simulink model "Position_Control_Test_SLAM_3LM"  (R2018b)
settings: Solver=VariableStepAuto  StartTime=0.0  StopTime=30  RelTol=1e-3
undefined symbols (not defined in the file): psi, quad, x, y, z
libraries: simulink x7, NLGCToolbox x6, shared6dof x1, aerolibnav x1
settings Model: Creator=hoang  LastModifiedBy=hoang
settings SFSimCC: SimUseLocalCustomCode=off
settings RTWCC: RTWUseLocalCustomCode=off

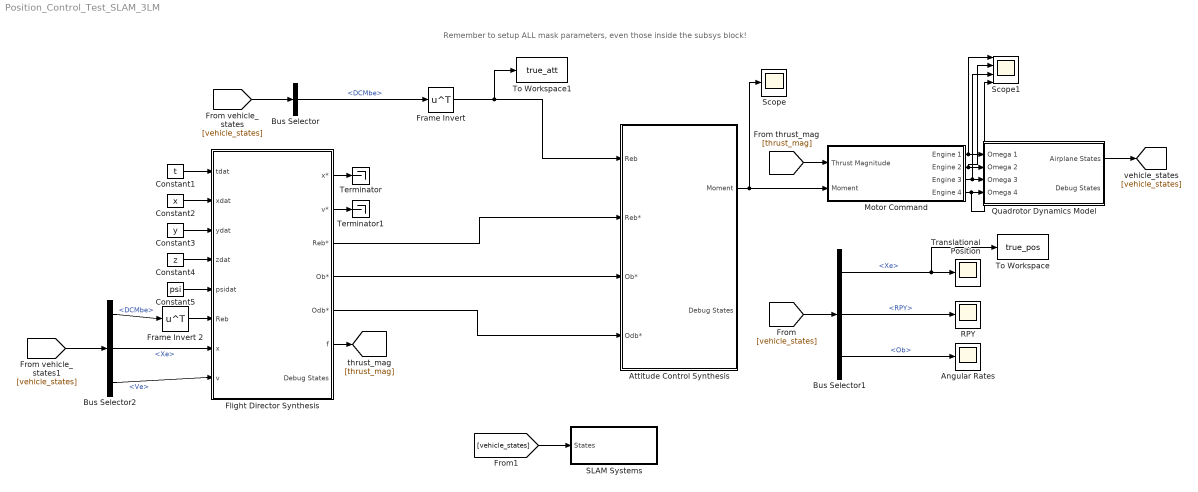
== system Position_Control_Test_SLAM_3LM ==
  note: Remember to setup ALL mask parameters, even those inside the subsys block!
  Angular Rates : Scope
  Attitude Control Synthesis : Subsystem  mask{quadrotor=quad, Ts1=1/120, kr=12, ko=4, Ts=0}
      mask prompts: quadrotor "Quadrotor Parameters"; Ts1 "Sampling Time"; kr "Attitude error gain (Kr)"; ko "Angular velocity error gain (Ko)"; Ts "Sampling Time (Ts)"
      settings: OpenFcn=set_param(gcbh,'LinkStatus','none');
  Bus Selector : BusSelector  OutputSignals=DCMbe
  Bus Selector1 : BusSelector  OutputSignals=Xe,RPY,Ob
  Bus Selector2 : BusSelector  OutputSignals=DCMbe,Xe,Ve
  Constant1 : Constant  Value=t
  Constant2 : Constant  Value=x
  Constant3 : Constant  Value=y
  Constant4 : Constant  Value=z
  Constant5 : Constant  Value=psi
  Flight Director Synthesis : Subsystem  mask{Ts=1/120, kx=64, kv=42, xinit=[0;0;-4], quadrotor=quad}
      mask prompts: Ts "Sampling Time (Ts)"; kx "Position Control Gain (kx)"; kv "Velocity Control Gain (kv)"; xinit "Initial position"; quadrotor "Quadrotor parameters"
      settings: OpenFcn=set_param(gcbh,'LinkStatus','none');
  Frame Invert : Math  Operator=transpose  SaturateOnIntegerOverflow=on
  Frame Invert 2 : Math  Operator=transpose  SaturateOnIntegerOverflow=on
  Motor Command : Subsystem  mask{quadrotor=quad}
      mask prompts: quadrotor "Quadrotor parameters"
      settings: OpenFcn=set_param(gcbh,'LinkStatus','none');
  Quadrotor Dynamics Model : Subsystem  AncestorBlock=NLGCToolbox/Quadrotor Dynamics Model  mask{xinit=[0;0;-4], quadrotor=quad}
      mask prompts: xinit "Initial Position [X,Y,Z]"; quadrotor "Quadrotor Model Struct"
  RPY : Scope
  SLAM Systems : Subsystem
  Scope : Scope
  Scope1 : Scope  NumInputPorts=4
  Terminator : Terminator
  Terminator1 : Terminator
  To Workspace : ToWorkspace  VariableName=true_pos  SaveFormat=Timeseries  SampleTime=-1
  To Workspace1 : ToWorkspace  VariableName=true_att  SaveFormat=Timeseries  SampleTime=-1
  Translational Position : Scope
  wires:
  Motor Command/1(Engine 1) -> Scope1/1, Quadrotor Dynamics Model/1(Omega 1)
  Motor Command/2(Engine 2) -> Scope1/2, Quadrotor Dynamics Model/2(Omega 2)
  Motor Command/3(Engine 3) -> Scope1/3, Quadrotor Dynamics Model/3(Omega 3)
  Motor Command/4(Engine 4) -> Scope1/4, Quadrotor Dynamics Model/4(Omega 4)
  Quadrotor Dynamics Model/1(Airplane States) -> [vehicle_states]
  [vehicle_states] -> Bus Selector/1
  Bus Selector/1 -> Frame Invert/1  "<DCMbe>"
  Frame Invert/1 -> To Workspace1/1, Attitude Control Synthesis/1(Reb)
  Flight Director Synthesis/3(Reb*) -> Attitude Control Synthesis/2(Reb*)
  Flight Director Synthesis/4(Ob*) -> Attitude Control Synthesis/3(Ob*)
  [vehicle_states] -> Bus Selector1/1
  Bus Selector1/2 -> RPY/1  "<RPY>"
  Bus Selector1/3 -> Angular Rates/1  "<Ob>"
  Bus Selector1/1 -> To Workspace/1, Translational Position/1  "<Xe>"
  Attitude Control Synthesis/1(Moment) -> Scope/1, Motor Command/2(Moment)
  Constant1/1 -> Flight Director Synthesis/1(tdat)
  Constant2/1 -> Flight Director Synthesis/2(xdat)
  Constant3/1 -> Flight Director Synthesis/3(ydat)
  Constant4/1 -> Flight Director Synthesis/4(zdat)
  Constant5/1 -> Flight Director Synthesis/5(psidat)
  [vehicle_states] -> Bus Selector2/1
  Frame Invert 2/1 -> Flight Director Synthesis/6(Reb)
  Bus Selector2/1 -> Frame Invert 2/1  "<DCMbe>"
  Bus Selector2/2 -> Flight Director Synthesis/7(x)  "<Xe>"
  Bus Selector2/3 -> Flight Director Synthesis/8(v)  "<Ve>"
  Flight Director Synthesis/5(Odb*) -> Attitude Control Synthesis/4(Odb*)
  Flight Director Synthesis/1(x*) -> Terminator/1
  Flight Director Synthesis/2(v*) -> Terminator1/1
  Flight Director Synthesis/6(f) -> [thrust_mag]
  [thrust_mag] -> Motor Command/1(" Thrust Magnitude")
  [vehicle_states] -> SLAM Systems/1(States)

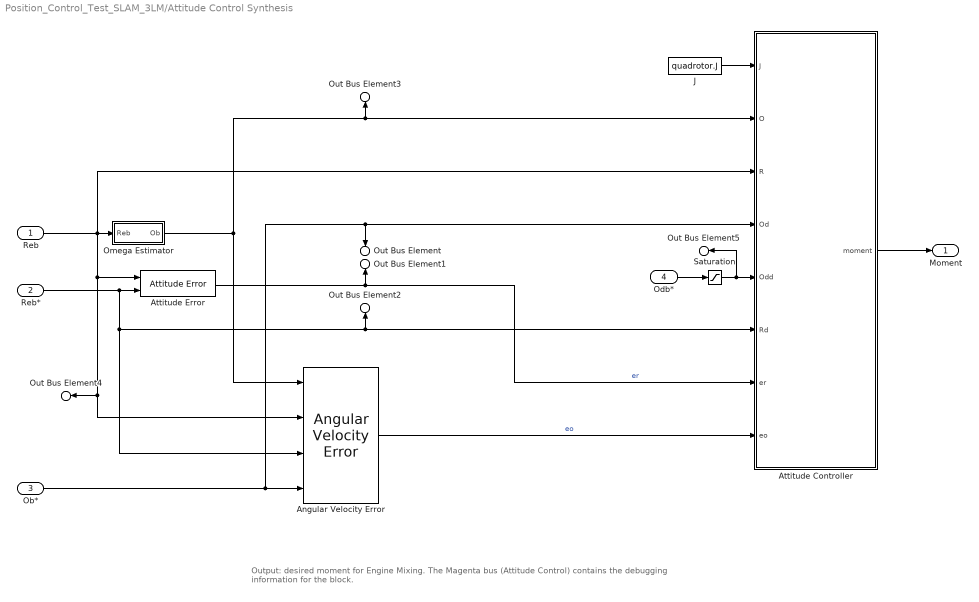
== system Position_Control_Test_SLAM_3LM/Attitude Control Synthesis ==
  note: Output: desired moment for Engine Mixing. The Magenta bus (Attitude Control) contains the debugging information for the block.
  Reb : Inport
  Reb* : Inport  Port=2
  Ob* : Inport  Port=3
  Odb* : Inport  Port=4
  Angular Velocity Error : NLGCToolbox/Angular Velocity Error  SystemSampleTime=-1
      settings: SourceProductName=Thinh - NLGC for Quadrotor
  Attitude Controller : MATLAB Function  TreatAsAtomicUnit=on
  Attitude Error : NLGCToolbox/Attitude Error  SystemSampleTime=-1
      settings: SourceProductName=Thinh - NLGC for Quadrotor
  J : Constant  Value=quadrotor.J
  Omega Estimator : Subsystem  mask{Ts=Ts1}
      mask prompts: Ts "Sampling Time (Ts)"
      settings: OpenFcn=set_param(gcbh,'LinkStatus','none');
  Saturation : Saturate  UpperLimit=1  LowerLimit=-1
  Moment : Outport
  Out Bus Element : Outport  Port=2  PortName=Debug States  Element=Ob*
  Out Bus Element1 : Outport  Port=2  PortName=Debug States  Element=er
  Out Bus Element2 : Outport  Port=2  PortName=Debug States  Element=Reb*
  Out Bus Element3 : Outport  Port=2  PortName=Debug States  Element=Ob
  Out Bus Element4 : Outport  Port=2  PortName=Debug States  Element=Reb
  Out Bus Element5 : Outport  Port=2  PortName=Debug States  Element=Odb*
  wires:
  Attitude Error/1 -> Out Bus Element1/1, Attitude Controller/7(er)  "er"
  Omega Estimator/1(Ob) -> Angular Velocity Error/1, Out Bus Element3/1, Attitude Controller/2(O)
  Angular Velocity Error/1 -> Attitude Controller/8(eo)  "eo"
  Saturation/1 -> Attitude Controller/5(Odd), Out Bus Element5/1
  Ob*/1 -> Angular Velocity Error/4, Attitude Controller/4(Od), Out Bus Element/1
  Reb*/1 -> Attitude Error/2, Angular Velocity Error/3, Attitude Controller/6(Rd), Out Bus Element2/1
  J/1 -> Attitude Controller/1(J)
  Attitude Controller/1(moment) -> Moment/1
  Odb*/1 -> Saturation/1
  Reb/1 -> Omega Estimator/1(Reb), Attitude Error/1, Angular Velocity Error/2, Out Bus Element4/1, Attitude Controller/3(R)

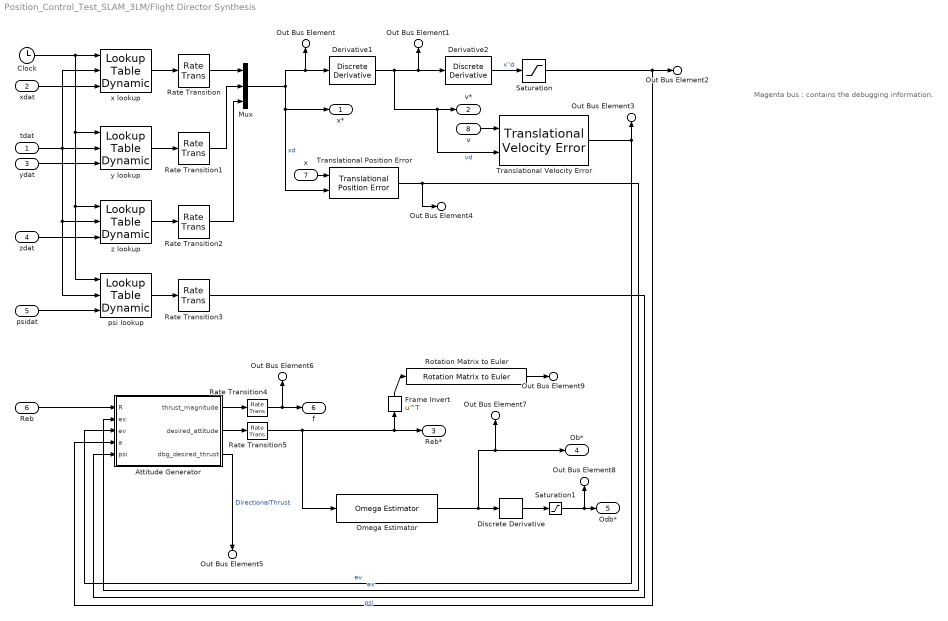
== system Position_Control_Test_SLAM_3LM/Flight Director Synthesis ==
  note: Magenta bus : contains the debugging information.
  tdat : Inport
  xdat : Inport  Port=2
  ydat : Inport  Port=3
  zdat : Inport  Port=4
  psidat : Inport  Port=5
  Reb : Inport  Port=6
  x : Inport  Port=7
  v : Inport  Port=8
  Attitude Generator : MATLAB Function  TreatAsAtomicUnit=on
  Clock : Clock
  Derivative1 : simulink/Discrete/Discrete Derivative  gainval=1.0  ICPrevScaledInput=xinit/Ts  OutMin=[]  OutMax=[]  OutDataType=fixdt(1, 16)  OutScaling=2^-10  DoSatur=off
  Derivative2 : simulink/Discrete/Discrete Derivative  gainval=1.0  ICPrevScaledInput=0.0  OutMin=[]  OutMax=[]  OutDataType=fixdt(1, 16)  OutScaling=2^-10  DoSatur=off
  Discrete Derivative : simulink/Discrete/Discrete Derivative  gainval=1.0  ICPrevScaledInput=0.0  OutMin=[]  OutMax=[]  OutDataType=fixdt(1, 16)  OutScaling=2^-10  DoSatur=off
  Frame Invert : Math  Operator=transpose  SaturateOnIntegerOverflow=on
  Mux : Mux  Inputs=3
  Omega Estimator : NLGCToolbox/Omega Estimator  Ts=Ts
      settings: SourceProductName=Thinh - NLGC for Quadrotor
  Rate Transition{,1..5} (6 alike) : RateTransition  OutPortSampleTime=Ts
  Rotation Matrix to Euler : NLGCToolbox/Rotation Matrix to Euler  SystemSampleTime=-1
      settings: SourceProductName=Thinh - NLGC for Quadrotor
  Saturation : Saturate  UpperLimit=1  LowerLimit=-1
  Saturation1 : Saturate  UpperLimit=1  LowerLimit=-1
  Translational Position Error : NLGCToolbox/Translational Position Error  SystemSampleTime=-1
      settings: SourceProductName=Thinh - NLGC for Quadrotor
  Translational Velocity Error : NLGCToolbox/Translational Velocity Error  SystemSampleTime=-1
      settings: SourceProductName=Thinh - NLGC for Quadrotor
  psi lookup : simulink/Lookup Tables/Lookup Table Dynamic  LookUpMeth=Interpolation-Use End Values  OutDataType=fixdt('double')  OutScaling=[]  OutputDataTypeScalingMode=Specify via dialog  OutDataTypeStr=double  DoSatur=off
      settings: SourceProductName=Simulink
  x lookup : simulink/Lookup Tables/Lookup Table Dynamic  LookUpMeth=Interpolation-Use End Values  OutDataType=fixdt('double')  OutScaling=[]  OutputDataTypeScalingMode=Specify via dialog  OutDataTypeStr=double  DoSatur=off
      settings: SourceProductName=Simulink
  y lookup : simulink/Lookup Tables/Lookup Table Dynamic  LookUpMeth=Interpolation-Use End Values  OutDataType=fixdt('double')  OutScaling=[]  OutputDataTypeScalingMode=Specify via dialog  OutDataTypeStr=double  DoSatur=off
      settings: SourceProductName=Simulink
  z lookup : simulink/Lookup Tables/Lookup Table Dynamic  LookUpMeth=Interpolation-Use End Values  OutDataType=fixdt('double')  OutScaling=[]  OutputDataTypeScalingMode=Specify via dialog  OutDataTypeStr=double  DoSatur=off
      settings: SourceProductName=Simulink
  x* : Outport
  v* : Outport  Port=2
  Reb* : Outport  Port=3
  Ob* : Outport  Port=4
  Odb* : Outport  Port=5
  f : Outport  Port=6
  Out Bus Element : Outport  Port=7  PortName=Debug States  Element=xd
  Out Bus Element1 : Outport  Port=7  PortName=Debug States  Element=vd
  Out Bus Element2 : Outport  Port=7  PortName=Debug States  Element=x''d
  Out Bus Element3 : Outport  Port=7  PortName=Debug States  Element=ev
  Out Bus Element4 : Outport  Port=7  PortName=Debug States  Element=ex
  Out Bus Element5 : Outport  Port=7  PortName=Debug States  Element=DirectionalThrust
  Out Bus Element6 : Outport  Port=7  PortName=Debug States  Element=DesiredThrust
  Out Bus Element7 : Outport  Port=7  PortName=Debug States  Element=DesiredOmega
  Out Bus Element8 : Outport  Port=7  PortName=Debug States  Element=Desired Angular Acceleration
  Out Bus Element9 : Outport  Port=7  PortName=Debug States  Element=RPY*
  wires:
  Frame Invert/1 -> Rotation Matrix to Euler/1
  Rotation Matrix to Euler/1 -> Out Bus Element9/1
  Saturation1/1 -> Out Bus Element8/1, Odb*/1
  Attitude Generator/3(dbg_desired_thrust) -> Out Bus Element5/1  "DirectionalThrust"
  Omega Estimator/1 -> Out Bus Element7/1, Ob*/1, Discrete Derivative/1
  v/1 -> Translational Velocity Error/1
  psidat/1 -> psi lookup/3
  Translational Velocity Error/1 -> Out Bus Element3/1, Attitude Generator/3(ev)  "ev"
  Translational Position Error/1 -> Attitude Generator/2(ex), Out Bus Element4/1  "ex"
  x/1 -> Translational Position Error/1
  Mux/1 -> Out Bus Element/1, Derivative1/1, Translational Position Error/2, x*/1  "xd"
  Rate Transition4/1 -> Out Bus Element6/1, f/1
  Rate Transition5/1 -> Frame Invert/1, Reb*/1, Omega Estimator/1
  Discrete Derivative/1 -> Saturation1/1
  Reb/1 -> Attitude Generator/1(R)
  Attitude Generator/2(desired_attitude) -> Rate Transition5/1
  Attitude Generator/1(thrust_magnitude) -> Rate Transition4/1
  Rate Transition3/1 -> Attitude Generator/5(psi)  "psi"
  Derivative2/1 -> Saturation/1  "x''d"
  psi lookup/1 -> Rate Transition3/1
  Derivative1/1 -> v*/1, Translational Velocity Error/2, Out Bus Element1/1, Derivative2/1  "vd"
  Rate Transition2/1 -> Mux/3
  Rate Transition1/1 -> Mux/2
  Rate Transition/1 -> Mux/1
  z lookup/1 -> Rate Transition2/1
  y lookup/1 -> Rate Transition1/1
  x lookup/1 -> Rate Transition/1
  zdat/1 -> z lookup/3
  ydat/1 -> y lookup/3
  xdat/1 -> x lookup/3
  Clock/1 -> x lookup/1, y lookup/1, z lookup/1, psi lookup/1
  tdat/1 -> y lookup/2, x lookup/2, z lookup/2, psi lookup/2
  Saturation/1 -> Attitude Generator/4(a), Out Bus Element2/1

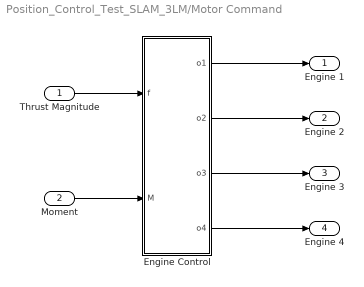
== system Position_Control_Test_SLAM_3LM/Motor Command ==
  " Thrust Magnitude" : Inport
  Moment : Inport  Port=2
  Engine Control : MATLAB Function  TreatAsAtomicUnit=on
  Engine 1 : Outport
  Engine 2 : Outport  Port=2
  Engine 3 : Outport  Port=3
  Engine 4 : Outport  Port=4
  wires:
  Engine Control/4(o4) -> Engine 4/1
  Engine Control/3(o3) -> Engine 3/1
  Engine Control/2(o2) -> Engine 2/1
  Engine Control/1(o1) -> Engine 1/1
  Moment/1 -> Engine Control/2(M)
  " Thrust Magnitude"/1 -> Engine Control/1(f)

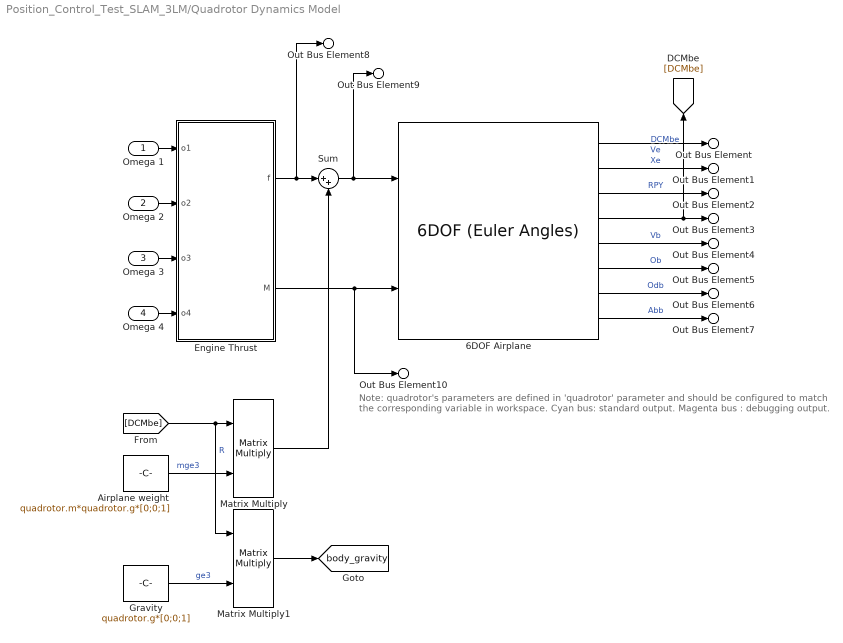
== system Position_Control_Test_SLAM_3LM/Quadrotor Dynamics Model ==
  note: Note: quadrotor's parameters are defined in 'quadrotor' parameter and should be configured to match the corresponding variable in workspace.
      | Cyan bus: standard output.
      | Magenta bus : debugging output.
  Omega 1 : Inport
  Omega 2 : Inport  Port=2
  Omega 3 : Inport  Port=3
  Omega 4 : Inport  Port=4
  6DOF Airplane : shared6dof/6DOF (Euler Angles)  units=Metric (MKS)  mtype=Fixed  rep=Euler Angles  xme_0=xinit  Vm_0=[0 0 0]  eul_0=[0 0 0]  pm_0=[0 0 0]  mass_0=quad.m  mass_e=0.5  mass_f=2.0  inertia=quad.J  inertia_e=eye(3)  inertia_f=2*eye(3)  k_quat=1.0  vre_flag=on  abi_flag=off  aMode=aMode  xme_statename=''  Vm_statename=''  eul_statename=''  quat_statename=''  pm_statename=''  mass_statename=''
      settings: SourceProductBaseCode=AE
  Airplane weight : Constant  Value=quadrotor.m*quadrotor.g*[0;0;1]
  Engine Thrust : MATLAB Function  TreatAsAtomicUnit=on
  Gravity : Constant  Value=quadrotor.g*[0;0;1]
  Matrix Multiply : Product  Multiplication=Matrix(*)
  Matrix Multiply1 : Product  Multiplication=Matrix(*)
  Sum : Sum  Inputs=|++
  Out Bus Element : Outport  PortName=Airplane States  Element=Ve
  Out Bus Element1 : Outport  PortName=Airplane States  Element=Xe
  Out Bus Element2 : Outport  PortName=Airplane States  Element=RPY
  Out Bus Element3 : Outport  PortName=Airplane States  Element=DCMbe
  Out Bus Element4 : Outport  PortName=Airplane States  Element=Vb
  Out Bus Element5 : Outport  PortName=Airplane States  Element=Ob
  Out Bus Element6 : Outport  PortName=Airplane States  Element=Odb
  Out Bus Element7 : Outport  PortName=Airplane States  Element=Abb
  Out Bus Element8 : Outport  Port=2  PortName=Debug States  Element=Thrust
  Out Bus Element9 : Outport  Port=2  PortName=Debug States  Element=Total Force
  Out Bus Element10 : Outport  Port=2  PortName=Debug States  Element=Moment
  tag scope: body_gravity=global
  wires:
  [DCMbe] -> Matrix Multiply1/1, Matrix Multiply/1  "R"
  Omega 1/1 -> Engine Thrust/1(o1)
  Omega 4/1 -> Engine Thrust/4(o4)
  Omega 3/1 -> Engine Thrust/3(o3)
  Omega 2/1 -> Engine Thrust/2(o2)
  Sum/1 -> 6DOF Airplane/1, Out Bus Element9/1
  Engine Thrust/2(M) -> 6DOF Airplane/2, Out Bus Element10/1
  6DOF Airplane/8 -> Out Bus Element7/1  "Abb"
  6DOF Airplane/5 -> Out Bus Element4/1  "Vb"
  6DOF Airplane/7 -> Out Bus Element6/1  "Odb"
  6DOF Airplane/2 -> Out Bus Element1/1  "Xe"
  6DOF Airplane/4 -> [DCMbe], Out Bus Element3/1  "DCMbe"
  6DOF Airplane/3 -> Out Bus Element2/1  "RPY"
  6DOF Airplane/1 -> Out Bus Element/1  "Ve"
  Matrix Multiply/1 -> Sum/2
  Engine Thrust/1(f) -> Sum/1, Out Bus Element8/1
  Airplane weight/1 -> Matrix Multiply/2  "mge3"
  6DOF Airplane/6 -> Out Bus Element5/1  "Ob"
  Gravity/1 -> Matrix Multiply1/2  "ge3"
  Matrix Multiply1/1 -> [body_gravity]

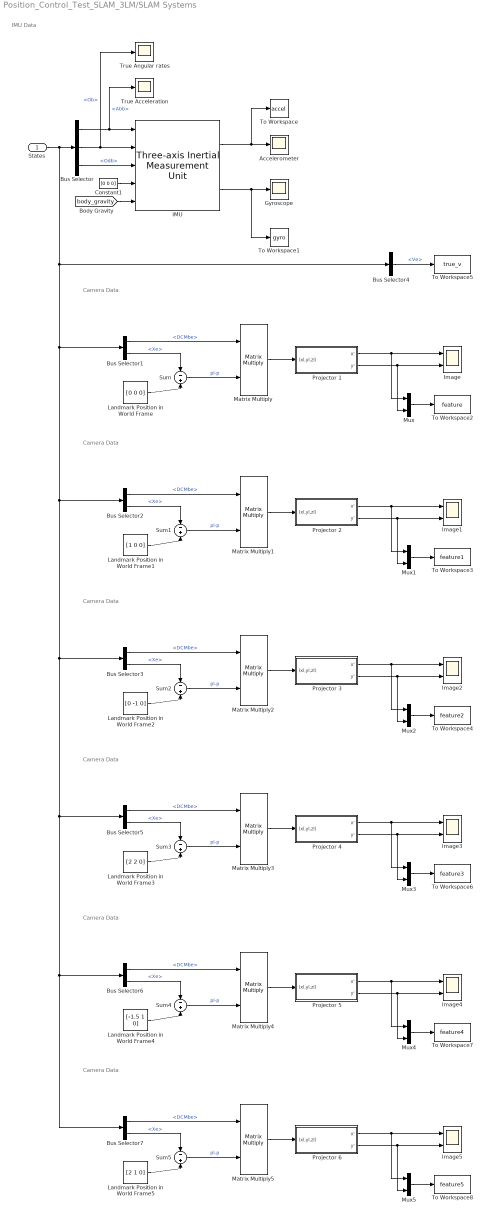
== system Position_Control_Test_SLAM_3LM/SLAM Systems ==
  note: Camera Data
  note: IMU Data
  note: Camera Data
  note: Camera Data
  note: Camera Data
  note: Camera Data
  note: Camera Data
  States : Inport
  Accelerometer : Scope
  Bus Selector : BusSelector  OutputSignals=Abb,Ob,Odb
  Bus Selector{1..3,5..7} (6 alike) : BusSelector  OutputSignals=DCMbe,Xe
  Bus Selector4 : BusSelector  OutputSignals=Ve
  Constant1 : Constant  Value=[0 0 0]
  Gyroscope : Scope
  IMU : aerolibnav/Three-axis Inertial Measurement Unit  units=Metric (MKS)  imu=[0 0 0]  i_Ts=0  dtype_a=off  w_a=190  z_a=0.707  a_sf_cc=[1 0 0; 0 1 0; 0 0 1]  a_bias=[0 0 0]  a_sat="[-inf  -inf  -inf  inf inf inf]"  dtype_g=off  w_g=190  z_g=0.707  g_sf_cc=[1 0 0; 0 1 0; 0 0 1]  g_bias=[0 0 0]  g_sens=[0 0 0]  g_sat="[-inf  -inf  -inf  inf inf inf]"  i_rand=off  i_seeds=[23093 23094 23095 23096 23097 23098]  i_pow=[0.001 0.001 0.001 0.0001 0.0001 0.0001]
  Image{,1..5} (6 alike) : Scope  NumInputPorts=2
  Landmark Position in World Frame : Constant  Value=[0 0 0]
  Landmark Position in World Frame1 : Constant  Value=[1 0 0]
  Landmark Position in World Frame2 : Constant  Value=[0 -1 0]
  Landmark Position in World Frame3 : Constant  Value=[2 2 0]
  Landmark Position in World Frame4 : Constant  Value=[-1.5 1 0]
  Landmark Position in World Frame5 : Constant  Value=[2 1 0]
  Matrix Multiply{,1..5} (6 alike) : Product  Multiplication=Matrix(*)
  Mux{,1..5} (6 alike) : Mux  Inputs=2
  Projector 1 : Subsystem
  Projector 2 : Subsystem
  Projector 3 : Subsystem
  Projector 4 : Subsystem
  Projector 5 : Subsystem
  Projector 6 : Subsystem
  Sum{,1..5} (6 alike) : Sum  Inputs=-+
  To Workspace : ToWorkspace  VariableName=accel  SaveFormat=Timeseries  SampleTime=-1
  To Workspace1 : ToWorkspace  VariableName=gyro  SaveFormat=Timeseries  SampleTime=-1
  To Workspace2 : ToWorkspace  VariableName=feature  SaveFormat=Timeseries  SampleTime=-1
  To Workspace3 : ToWorkspace  VariableName=feature1  SaveFormat=Timeseries  SampleTime=-1
  To Workspace4 : ToWorkspace  VariableName=feature2  SaveFormat=Timeseries  SampleTime=-1
  To Workspace5 : ToWorkspace  VariableName=true_v  SaveFormat=Timeseries  SampleTime=-1
  To Workspace6 : ToWorkspace  VariableName=feature3  SaveFormat=Timeseries  SampleTime=-1
  To Workspace7 : ToWorkspace  VariableName=feature4  SaveFormat=Timeseries  SampleTime=-1
  To Workspace8 : ToWorkspace  VariableName=feature5  SaveFormat=Timeseries  SampleTime=-1
  True Acceleration : Scope
  True Angular rates : Scope
  wires:
  Bus Selector/2 -> True Angular rates/1, IMU/2  "<Ob>"
  Bus Selector/3 -> IMU/3  "<Odb>"
  Bus Selector/1 -> True Acceleration/1, IMU/1  "<Abb>"
  IMU/1 -> To Workspace/1, Accelerometer/1
  Constant1/1 -> IMU/4
  IMU/2 -> To Workspace1/1, Gyroscope/1
  [body_gravity] -> IMU/5
  Bus Selector1/1 -> Matrix Multiply/1  "<DCMbe>"
  Landmark Position in World Frame/1 -> Sum/2
  Bus Selector1/2 -> Sum/1  "<Xe>"
  Sum/1 -> Matrix Multiply/2  "pl-p"
  Matrix Multiply/1 -> Projector 1/1((xl,yl,zl))
  Projector 1/2(y') -> Mux/2, Image/2
  Projector 1/1(x') -> Mux/1, Image/1
  Mux/1 -> To Workspace2/1
  Matrix Multiply1/1 -> Projector 2/1((xl,yl,zl))
  Landmark Position in World Frame1/1 -> Sum1/2
  Bus Selector2/1 -> Matrix Multiply1/1  "<DCMbe>"
  Projector 2/1(x') -> Mux1/1, Image1/1
  Mux1/1 -> To Workspace3/1
  Bus Selector2/2 -> Sum1/1  "<Xe>"
  Sum1/1 -> Matrix Multiply1/2  "pl-p"
  Projector 2/2(y') -> Mux1/2, Image1/2
  Projector 3/2(y') -> Image2/2, Mux2/2
  Sum2/1 -> Matrix Multiply2/2  "pl-p"
  Bus Selector3/2 -> Sum2/1  "<Xe>"
  Mux2/1 -> To Workspace4/1
  Projector 3/1(x') -> Image2/1, Mux2/1
  Bus Selector3/1 -> Matrix Multiply2/1  "<DCMbe>"
  Landmark Position in World Frame2/1 -> Sum2/2
  Matrix Multiply2/1 -> Projector 3/1((xl,yl,zl))
  Bus Selector4/1 -> To Workspace5/1  "<Ve>"
  Matrix Multiply3/1 -> Projector 4/1((xl,yl,zl))
  Landmark Position in World Frame3/1 -> Sum3/2
  Bus Selector5/1 -> Matrix Multiply3/1  "<DCMbe>"
  Projector 4/1(x') -> Mux3/1, Image3/1
  Mux3/1 -> To Workspace6/1
  Bus Selector5/2 -> Sum3/1  "<Xe>"
  Sum3/1 -> Matrix Multiply3/2  "pl-p"
  Projector 4/2(y') -> Mux3/2, Image3/2
  Projector 5/2(y') -> Image4/2, Mux4/2
  Sum4/1 -> Matrix Multiply4/2  "pl-p"
  Bus Selector6/2 -> Sum4/1  "<Xe>"
  Mux4/1 -> To Workspace7/1
  Projector 5/1(x') -> Image4/1, Mux4/1
  Bus Selector6/1 -> Matrix Multiply4/1  "<DCMbe>"
  Landmark Position in World Frame4/1 -> Sum4/2
  Matrix Multiply4/1 -> Projector 5/1((xl,yl,zl))
  Matrix Multiply5/1 -> Projector 6/1((xl,yl,zl))
  Landmark Position in World Frame5/1 -> Sum5/2
  Bus Selector7/1 -> Matrix Multiply5/1  "<DCMbe>"
  Projector 6/1(x') -> Mux5/1, Image5/1
  Mux5/1 -> To Workspace8/1
  Bus Selector7/2 -> Sum5/1  "<Xe>"
  Sum5/1 -> Matrix Multiply5/2  "pl-p"
  Projector 6/2(y') -> Mux5/2, Image5/2
  States/1 -> Bus Selector4/1, Bus Selector7/1, Bus Selector6/1, Bus Selector5/1, Bus Selector3/1, Bus Selector2/1, Bus Selector1/1, Bus Selector/1

== system Position_Control_Test_SLAM_3LM/Attitude Control Synthesis/Omega Estimator ==
  Reb : Inport
  Delay : Delay  DelayLength=1
  Omega Estimator : MATLAB Function  TreatAsAtomicUnit=on
  Rate Transition2 : RateTransition  InitialCondition=diag([1,1,1])  OutPortSampleTime=Ts
  Ob : Outport
  wires:
  Delay/1 -> Omega Estimator/1(Rd1)
  Reb/1 -> Rate Transition2/1
  Omega Estimator/1(Omega) -> Ob/1
  Rate Transition2/1 -> Delay/1, Omega Estimator/2(Rd2)

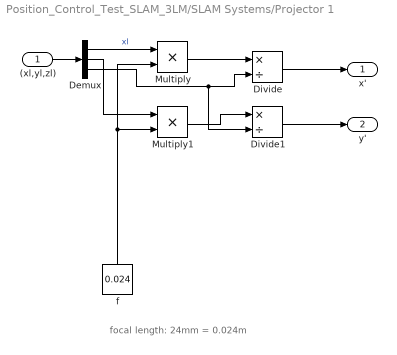
== system Position_Control_Test_SLAM_3LM/SLAM Systems/Projector 1 ==
  note: focal length: 24mm = 0.024m
  (xl,yl,zl) : Inport
  Demux : Demux  Outputs=3
  Divide : Product  Inputs=*/
  Divide1 : Product  Inputs=*/
  Multiply : Product
  Multiply1 : Product
  f : Constant  Value=0.024
  x' : Outport
  y' : Outport  Port=2
  wires:
  (xl,yl,zl)/1 -> Demux/1
  Demux/1 -> Multiply/1  "xl"
  f/1 -> Multiply1/2, Multiply/2
  Multiply/1 -> Divide/1
  Demux/3 -> Divide1/2, Divide/2
  Divide/1 -> x'/1
  Demux/2 -> Multiply1/1
  Multiply1/1 -> Divide1/1
  Divide1/1 -> y'/1

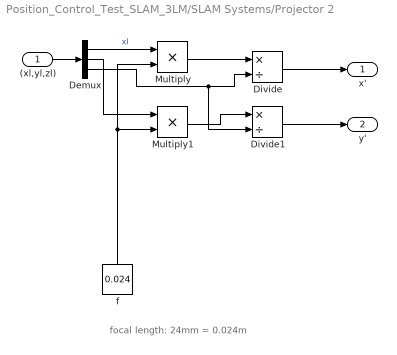
== system Position_Control_Test_SLAM_3LM/SLAM Systems/Projector 2 ==
  note: focal length: 24mm = 0.024m
  (xl,yl,zl) : Inport
  Demux : Demux  Outputs=3
  Divide : Product  Inputs=*/
  Divide1 : Product  Inputs=*/
  Multiply : Product
  Multiply1 : Product
  f : Constant  Value=0.024
  x' : Outport
  y' : Outport  Port=2
  wires:
  (xl,yl,zl)/1 -> Demux/1
  Demux/1 -> Multiply/1  "xl"
  f/1 -> Multiply1/2, Multiply/2
  Multiply/1 -> Divide/1
  Demux/3 -> Divide1/2, Divide/2
  Divide/1 -> x'/1
  Demux/2 -> Multiply1/1
  Multiply1/1 -> Divide1/1
  Divide1/1 -> y'/1

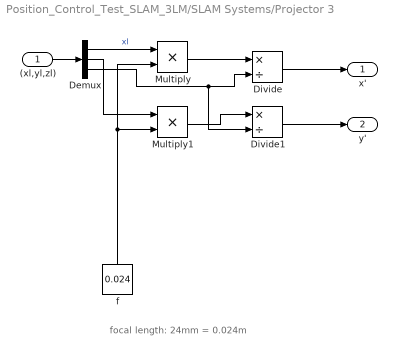
== system Position_Control_Test_SLAM_3LM/SLAM Systems/Projector 3 ==
  note: focal length: 24mm = 0.024m
  (xl,yl,zl) : Inport
  Demux : Demux  Outputs=3
  Divide : Product  Inputs=*/
  Divide1 : Product  Inputs=*/
  Multiply : Product
  Multiply1 : Product
  f : Constant  Value=0.024
  x' : Outport
  y' : Outport  Port=2
  wires:
  Divide1/1 -> y'/1
  Multiply1/1 -> Divide1/1
  Demux/2 -> Multiply1/1
  Divide/1 -> x'/1
  Demux/3 -> Divide/2, Divide1/2
  Multiply/1 -> Divide/1
  f/1 -> Multiply/2, Multiply1/2
  Demux/1 -> Multiply/1  "xl"
  (xl,yl,zl)/1 -> Demux/1

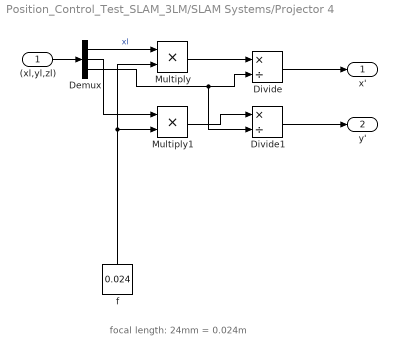
== system Position_Control_Test_SLAM_3LM/SLAM Systems/Projector 4 ==
  note: focal length: 24mm = 0.024m
  (xl,yl,zl) : Inport
  Demux : Demux  Outputs=3
  Divide : Product  Inputs=*/
  Divide1 : Product  Inputs=*/
  Multiply : Product
  Multiply1 : Product
  f : Constant  Value=0.024
  x' : Outport
  y' : Outport  Port=2
  wires:
  (xl,yl,zl)/1 -> Demux/1
  Demux/1 -> Multiply/1  "xl"
  f/1 -> Multiply1/2, Multiply/2
  Multiply/1 -> Divide/1
  Demux/3 -> Divide1/2, Divide/2
  Divide/1 -> x'/1
  Demux/2 -> Multiply1/1
  Multiply1/1 -> Divide1/1
  Divide1/1 -> y'/1

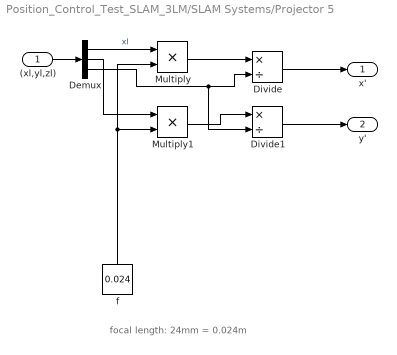
== system Position_Control_Test_SLAM_3LM/SLAM Systems/Projector 5 ==
  note: focal length: 24mm = 0.024m
  (xl,yl,zl) : Inport
  Demux : Demux  Outputs=3
  Divide : Product  Inputs=*/
  Divide1 : Product  Inputs=*/
  Multiply : Product
  Multiply1 : Product
  f : Constant  Value=0.024
  x' : Outport
  y' : Outport  Port=2
  wires:
  Divide1/1 -> y'/1
  Multiply1/1 -> Divide1/1
  Demux/2 -> Multiply1/1
  Divide/1 -> x'/1
  Demux/3 -> Divide/2, Divide1/2
  Multiply/1 -> Divide/1
  f/1 -> Multiply/2, Multiply1/2
  Demux/1 -> Multiply/1  "xl"
  (xl,yl,zl)/1 -> Demux/1

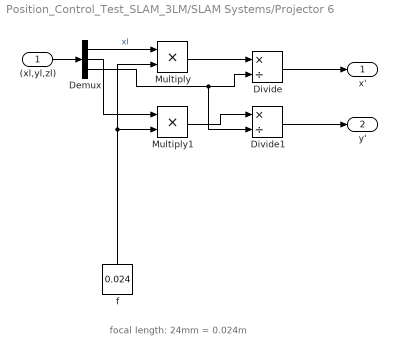
== system Position_Control_Test_SLAM_3LM/SLAM Systems/Projector 6 ==
  note: focal length: 24mm = 0.024m
  (xl,yl,zl) : Inport
  Demux : Demux  Outputs=3
  Divide : Product  Inputs=*/
  Divide1 : Product  Inputs=*/
  Multiply : Product
  Multiply1 : Product
  f : Constant  Value=0.024
  x' : Outport
  y' : Outport  Port=2
  wires:
  (xl,yl,zl)/1 -> Demux/1
  Demux/1 -> Multiply/1  "xl"
  f/1 -> Multiply1/2, Multiply/2
  Multiply/1 -> Divide/1
  Demux/3 -> Divide1/2, Divide/2
  Divide/1 -> x'/1
  Demux/2 -> Multiply1/1
  Multiply1/1 -> Divide1/1
  Divide1/1 -> y'/1

== matlab function Position_Control_Test_SLAM_3LM/Flight Director Synthesis/Attitude Generator ==
  data: R input size=[3 3]; thrust_magnitude output size=1; ex input size=[3 1]; ev input size=[3 1]; a input size=[3 1]; psi input size=1; desired_attitude output size=[3 3]; kx parameter; kv parameter; quadrotor parameter; dbg_desired_thrust output
function [thrust_magnitude,desired_attitude,dbg_desired_thrust] = fcn(R,ex,ev,a,psi,kx,kv,quadrotor) % R: b->i

e3 = [0 0 1]';

if (norm(a)>100) % Fuse for large intial derivatives
    a = [0;0;0];
end 

desired_thrust = - kx*ex - kv*ev - quadrotor.m*quadrotor.g*e3 + quadrotor.m*a;
dbg_desired_thrust = desired_thrust;

% Desired Attitude Calculation
z_direction = -desired_thrust/norm(desired_thrust); % b3, from [0 0 1]'
x_direction = findDirection(psi, z_direction); % b1, from [1 0 0]'
y_direction = hat(z_direction)*x_direction; % b2, from [0 1 0]'
desired_attitude = trnorm([x_direction y_direction z_direction]); % b->i, since R[1 0 0]' = x_direction => RI = R, thus it eats a body vector and returns an inertial vector

thrust_magnitude = norm(desired_thrust) * (e3'*R'*desired_attitude*e3);

end

% Function to find Promoted Direction Vector
function y = findDirection(psi,thrust_direction)
Rpsi = mod_rpy2r(0,0,psi); % b->i
ddv = Rpsi*[1 0 0]'; % Provisional Desired Direction Vector (DDV)
pdv = - (hat(thrust_direction) * (hat(thrust_direction) * ddv)); % Promoted Direction Vector (PDV)
y = pdv/norm(pdv);
end

== matlab function Position_Control_Test_SLAM_3LM/Attitude Control Synthesis/Attitude Controller ==
  data: J input size=[3 3]; moment output size=[3 1]; O input size=[3 1]; R input size=[3 3]; Od input size=[3 1]; Odd input size=[3 1]; Rd input size=[3 3]; er input size=[3 1]; eo input size=[3 1]; kr parameter; ko parameter
function moment = fcn(J,O,R,Od,Odd,Rd,er,eo,kr, ko)
moment = nlgc_moment(J,O,R,Od,Odd,Rd,er,eo,kr,ko);

== matlab function Position_Control_Test_SLAM_3LM/Motor Command/Engine Control ==
  data: f input size=1; o1 output size=1; M input size=[3 1]; o2 output size=1; o3 output size=1; o4 output size=1; quadrotor parameter
function [o1,o2,o3,o4] = fcn(f,M,quadrotor)
[o1,o2,o3,o4] = engine_mix(f,M,quadrotor.ct,quadrotor.dctcq);

== matlab function Position_Control_Test_SLAM_3LM/Attitude Control Synthesis/Omega Estimator/Omega Estimator ==
  data: Rd1 input size=[3 3]; Omega output size=[3 1]; Rd2 input size=[3 3]; Ts parameter
function Omega = fcn(Rd1,Rd2,Ts)
Omega = rr2ar(Rd1,Rd2,Ts);
% Omega=OmegaP;
end

== matlab function Position_Control_Test_SLAM_3LM/Quadrotor Dynamics Model/Engine Thrust ==
  data: o1 input size=1; f output size=[3 1]; o2 input size=1; o3 input size=1; o4 input size=1; M output size=[3 1]; quadrotor parameter
function [f,M] = fcn(o1,o2,o3,o4,quadrotor)
[f,M] = omega2force(o1,o2,o3,o4,quadrotor.ct,quadrotor.dctcq);
